simulink model "controller_for_bicycle"  (R2021a)
settings: Solver=VariableStepAuto  StartTime=0.0  StopTime=10.0  RelTol=1e-3
values from neighbouring files (symbols this model uses):
  Fyf = zeros(1,57)    [FyfLookUpNewCar.m]    (also in Fyf_loopup_table.mat = [-9372.31873381 -9371.87234491 -9368.75632133 -9360.32413915)
  SlipAngle = -SlipAngle    [FyfLookUpNewCar.m]    (also in Fyf_loopup_table.mat = [0.153111393254 0.147643129209 0.142174865164 0.13670660112 )
libraries: simulink_extras x1, autolibshared x1, simulink x1
settings Model: Creator=chnwa  LastModifiedBy=chnwa

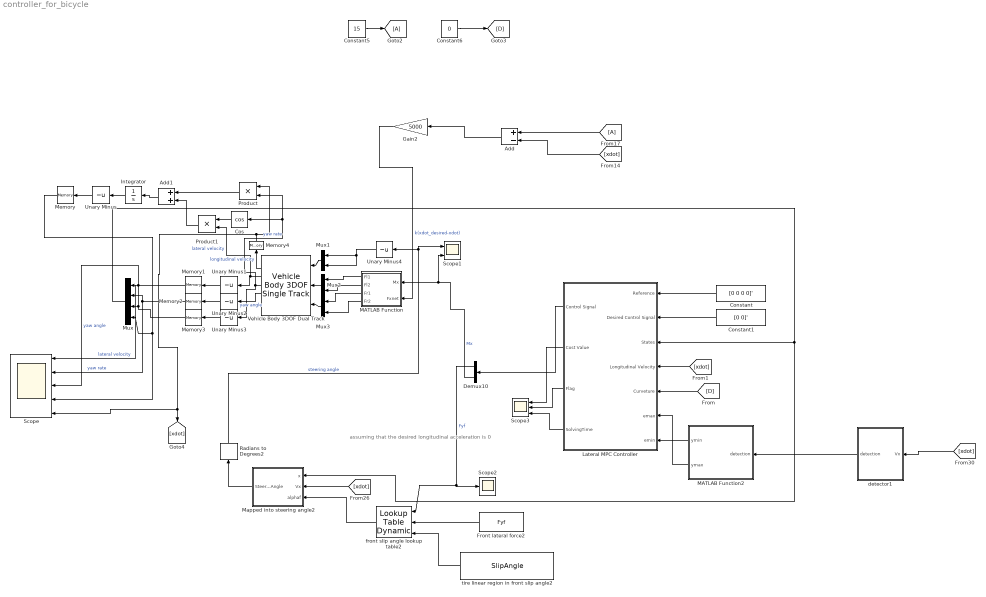
== system controller_for_bicycle ==
  note: assuming that the desired longitudinal acceleration is 0
  Add : Sum  Inputs=+-
  Add1 : Sum
  Constant : Constant  Value=[0 0 0 0]'
  Constant1 : Constant  Value=[0 0]'
  Constant5 : Constant  Value=15
  Constant6 : Constant  Value=0
  Cos : Trigonometry  Operator=cos
  Demux10 : Demux  Outputs=2
  Front lateral force2 : Constant  Value=Fyf
  Gain2 : Gain  Gain=5000
  Integrator : Integrator
  Lateral MPC Controller : Subsystem
  MATLAB Function : MATLAB Function  TreatAsAtomicUnit=on
  MATLAB Function2 : MATLAB Function  TreatAsAtomicUnit=on
  Mapped into steering angle2 : MATLAB Function  TreatAsAtomicUnit=on
  Memory{,1..3} (4 alike) : Memory
  Memory4 : Memory  InitialCondition=15
  Mux : Mux
  Mux1 : Mux  Inputs=2
  Mux2 : Mux  Inputs=2
  Mux3 : Mux  Inputs=2
  Product : Product
  Product1 : Product
  Radians to Degrees2 : simulink_extras/Transformations/Radians to Degrees
  Scope : Scope  NumInputPorts=5
  Scope1 : Scope  NumInputPorts=2
  Scope2 : Scope
  Scope3 : Scope  NumInputPorts=3
  Unary Minus{,1..4} (5 alike) : UnaryMinus
  Vehicle Body 3DOF Dual Track : autolibshared/Vehicle Body 3DOF Single Track  trackMode=Dual  inputMode=External longitudinal forces  frontSteerMode=on  rearSteerMode=off  windMode=off  muMode=off  extFMode=off  extMMode=off  htchFMode=off  htchMMode=off  extXo=off  extpsio=off  extxdoto=off  extro=off  extYo=off  extTamb=off  extydoto=off  aMode=2  NF=2  NR=2  m=2272  a=1.11  b=1.67  h=0.35  dh=1  hh=0.2  X_o=0  xdot_o=15  CalphaMode=off  sigmaMode=on  d=0  hl=0  w=[1.4,1.4]  Cy_f=1.822e5  Cy_r=1.822e5  sigma_f=.1  sigma_r=.1  alpha_f_brk=[-.1 .1]  Cy_f_data=[-9e3 9e3]  alpha_r_brk=[-.1 .1]  Cy_r_data=[-9e3 9e3]  Y_o=0  ydot_o=0  Izz=4600  psi_o=0  r_o=0  Af=2  Cd=.3  Cl=.1  Cpm=.1  beta_w=[0:0.01:0.3]  Cs=[0:0.03:0.9]  Cym=[0:0.01:0.3]  Pabs=101325  Tair=273  g=9.81  mu=0.7  xdot_tol=.01  Fznom=5000  Fxtire_sat=7e4  Fytire_sat=7e4  longOff=0  latOff=0  vertOff=0  wrapAng=off
      settings: SourceProductBaseCode=PW,DR,MT,UV,VE
  detector1 : Subsystem
  front slip angle lookup table2 : simulink/Lookup Tables/Lookup Table Dynamic  LookUpMeth=Interpolation-Use End Values  OutDataType=fixdt('double')  OutScaling=[]  OutputDataTypeScalingMode=Specify via dialog  OutDataTypeStr=double  DoSatur=off
  tire linear region in front slip angle2 : Constant  Value=SlipAngle
  wires:
  [xdot] -> Lateral MPC Controller/4(Longitudinal Velocity)
  tire linear region in front slip angle2/1 -> front slip angle lookup table2/3
  Memory3/1 -> Scope/3, Mux/3  "yaw angle"
  Constant/1 -> Lateral MPC Controller/1(Reference)
  Lateral MPC Controller/2(Cost Value) -> Scope3/1
  MATLAB Function/3(Fr1) -> Mux3/1
  [xdot] -> detector1/1(Vx)
  MATLAB Function2/2(ymax) -> Lateral MPC Controller/6(emax)
  Lateral MPC Controller/4(SolvingTime) -> Scope3/3
  front slip angle lookup table2/1 -> Mapped into steering angle2/3(alphaf)
  Lateral MPC Controller/3(Flag) -> Scope3/2
  Demux10/2 -> Scope1/2, MATLAB Function/1(Mx)  "Mx"
  Lateral MPC Controller/1(Control Signal) -> Demux10/1
  MATLAB Function/1(Fl1) -> Mux2/1
  MATLAB Function/2(Fl2) -> Mux2/2
  MATLAB Function/4(Fr2) -> Mux3/2
  Demux10/1 -> Scope2/1, front slip angle lookup table2/1  "Fyf"
  Gain2/1 -> MATLAB Function/2(Fxnet)  "k(xdot_desired-xdot)"
  Mux/1 -> Mapped into steering angle2/1(x), Lateral MPC Controller/3(States)
  [A] -> Add/1
  Radians to Degrees2/1 -> Unary Minus4/1, Scope1/1  "steering angle"
  [D] -> Lateral MPC Controller/5(Curveture)
  Memory2/1 -> Scope/2, Mux/2  "yaw rate"
  Mapped into steering angle2/1(SteeringAngle) -> Radians to Degrees2/1
  MATLAB Function2/1(ymin) -> Lateral MPC Controller/7(emin)
  [xdot] -> Mapped into steering angle2/2(Vx)
  [xdot] -> Add/2
  Front lateral force2/1 -> front slip angle lookup table2/2
  detector1/1(detection) -> MATLAB Function2/1(detection)
  Vehicle Body 3DOF Dual Track/2 -> Memory4/1  "longitudinal velocity"
  Add/1 -> Gain2/1
  Memory1/1 -> Scope/1, Mux/1  "lateral velocity"
  Constant1/1 -> Lateral MPC Controller/2(Desired Control Signal)
  Mux1/1 -> Vehicle Body 3DOF Dual Track/1
  Mux2/1 -> Vehicle Body 3DOF Dual Track/2
  Mux3/1 -> Vehicle Body 3DOF Dual Track/3
  Unary Minus/1 -> Memory/1
  Memory/1 -> Scope/4, Mux/4
  Unary Minus1/1 -> Memory1/1
  Vehicle Body 3DOF Dual Track/3 -> Product1/2, Unary Minus1/1  "lateral velocity"
  Unary Minus2/1 -> Memory2/1
  Vehicle Body 3DOF Dual Track/5 -> Unary Minus2/1  "yaw angle"
  Unary Minus3/1 -> Memory3/1
  Vehicle Body 3DOF Dual Track/4 -> Product/2, Cos/1, Unary Minus3/1  "yaw rate"
  Unary Minus4/1 -> Mux1/2, Mux1/1
  Constant5/1 -> [A]
  Constant6/1 -> [D]
  Cos/1 -> Product1/1
  Product/1 -> Add1/1
  Product1/1 -> Add1/2
  Add1/1 -> Integrator/1
  Integrator/1 -> Unary Minus/1
  Memory4/1 -> Product/1, [xdot], Scope/5

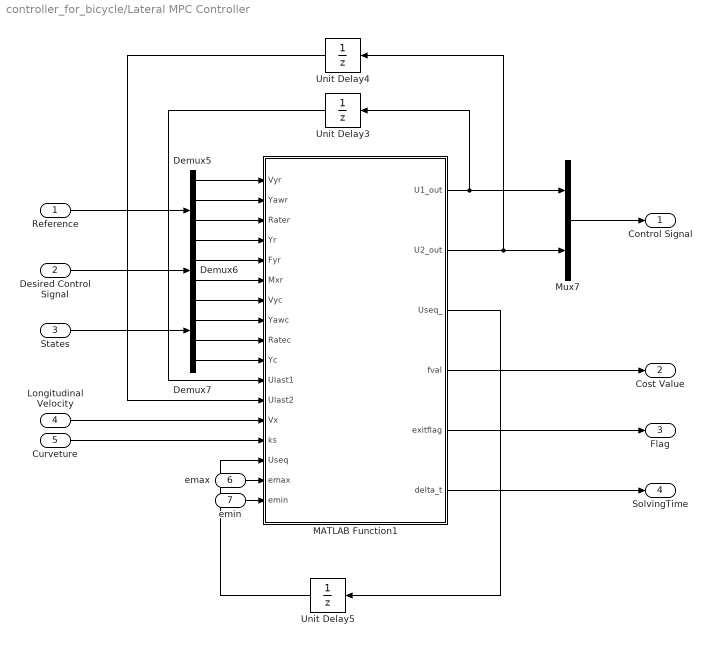
== system controller_for_bicycle/Lateral MPC Controller ==
  Reference : Inport
  Desired Control Signal : Inport  Port=2
  States : Inport  Port=3
  Longitudinal Velocity : Inport  Port=4
  Curveture : Inport  Port=5
  emax : Inport  Port=6
  emin : Inport  Port=7
  Demux5 : Demux
  Demux6 : Demux  Outputs=2
  Demux7 : Demux
  MATLAB Function1 : MATLAB Function  TreatAsAtomicUnit=on
  Mux7 : Mux  Inputs=2
  Unit Delay3 : UnitDelay  SampleTime=-1  HasFrameUpgradeWarning=on
  Unit Delay4 : UnitDelay  SampleTime=-1  HasFrameUpgradeWarning=on
  Unit Delay5 : UnitDelay  InitialCondition=zeros(31,2)  SampleTime=-1  HasFrameUpgradeWarning=on
  Control Signal : Outport
  Cost Value : Outport  Port=2
  Flag : Outport  Port=3
  SolvingTime : Outport  Port=4
  wires:
  Demux5/3 -> MATLAB Function1/3(Rater)
  Desired Control Signal/1 -> Demux6/1
  MATLAB Function1/5(exitflag) -> Flag/1
  MATLAB Function1/2(U2_out) -> Mux7/2, Unit Delay4/1
  Demux5/1 -> MATLAB Function1/1(Vyr)
  Unit Delay4/1 -> MATLAB Function1/12(Ulast2)
  Longitudinal Velocity/1 -> MATLAB Function1/13(Vx)
  Demux7/3 -> MATLAB Function1/9(Ratec)
  MATLAB Function1/3(Useq_) -> Unit Delay5/1
  Demux7/1 -> MATLAB Function1/7(Vyc)
  Demux5/4 -> MATLAB Function1/4(Yr)
  MATLAB Function1/4(fval) -> Cost Value/1
  Curveture/1 -> MATLAB Function1/14(ks)
  emax/1 -> MATLAB Function1/16(emax)
  MATLAB Function1/1(U1_out) -> Mux7/1, Unit Delay3/1
  Demux7/2 -> MATLAB Function1/8(Yawc)
  Demux7/4 -> MATLAB Function1/10(Yc)
  Reference/1 -> Demux5/1
  Mux7/1 -> Control Signal/1
  Unit Delay5/1 -> MATLAB Function1/15(Useq)
  Unit Delay3/1 -> MATLAB Function1/11(Ulast1)
  States/1 -> Demux7/1
  MATLAB Function1/6(delta_t) -> SolvingTime/1
  Demux6/2 -> MATLAB Function1/6(Mxr)
  Demux6/1 -> MATLAB Function1/5(Fyr)
  Demux5/2 -> MATLAB Function1/2(Yawr)
  emin/1 -> MATLAB Function1/17(emin)

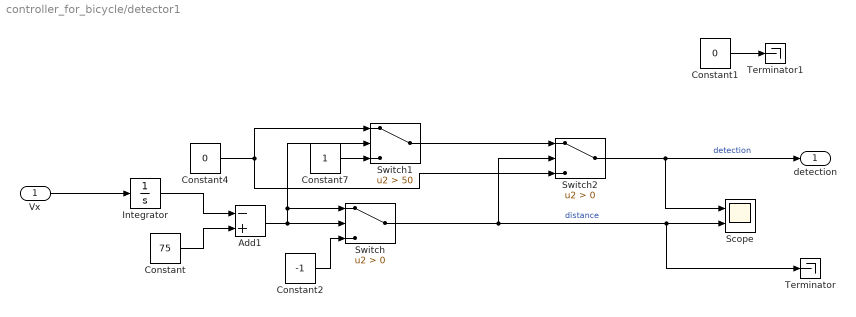
== system controller_for_bicycle/detector1 ==
  Vx : Inport
  Add1 : Sum  Inputs=-+
  Constant : Constant  Value=75
  Constant1 : Constant  Value=0
  Constant2 : Constant  Value=-1
  Constant4 : Constant  Value=0
  Constant7 : Constant
  Integrator : Integrator
  Scope : Scope  NumInputPorts=2
  Switch : Switch  Criteria=u2 > Threshold
  Switch1 : Switch  Criteria=u2 > Threshold  Threshold=50
  Switch2 : Switch  Criteria=u2 > Threshold
  Terminator : Terminator
  Terminator1 : Terminator
  detection : Outport
  wires:
  Constant2/1 -> Switch/3
  Constant4/1 -> Switch2/3, Switch1/1
  Vx/1 -> Integrator/1
  Integrator/1 -> Add1/1
  Switch/1 -> Switch2/2, Terminator/1, Scope/2  "distance"
  Constant7/1 -> Switch1/3
  Add1/1 -> Switch1/2, Switch/1, Switch/2
  Switch1/1 -> Switch2/1
  Constant/1 -> Add1/2
  Switch2/1 -> detection/1, Scope/1  "detection"
  Constant1/1 -> Terminator1/1

== matlab function controller_for_bicycle/MATLAB Function2 ==
  data: detection input; ymin output; ymax output
function [ymin,ymax] = fcn(detection)

% miu = 0.7; %frction cooeficient 0.7 for dry road and 0.4 for wet
% g = 9.81; % gravity
% m = 2272;   %mass
% lf = 1.11;  % distance from front axle to the mass center
% lr = 1.67;  % distance from rear axle to the mass center
% C_a = 1.822e5; % rear cornering stifness
% 
% Fz = m*g*lf/(lf+lr)/2; % the load that beared by the rear tire
% 
% rmax = g*miu/Vx; %max yaw rate
% threshold = atan(3*miu*Fz/C_a);
% 
% r = x(2);
% vmax = lr*r+Vx*threshold;   %max lateral velocity
% vmin = lr*r-Vx*threshold;   %min lateral velocity

if detection == 1
    ymin = 5;%50m is the distance from which obstacle is detected
    ymax = 10;
else
    ymin = -10;
    ymax = 10;
end

== matlab function controller_for_bicycle/Lateral MPC Controller/MATLAB Function1 ==
  data: Vyr input; U1_out output; Yawr input; Rater input; Yr input; Fyr input; Mxr input; Vyc input; Yawc input; Ratec input; Yc input; Ulast1 input; Ulast2 input; Vx input; ks input; Useq input; U2_out output; Useq_ output; fval output; exitflag output; delta_t output; emax input; emin input
function [U1_out,U2_out,Useq_,fval,exitflag,delta_t] = fcn(Vyr,Yawr,Rater,Yr, Fyr,Mxr,Vyc,Yawc,Ratec,Yc,Ulast1,Ulast2,Vx,ks,Useq,emax,emin)
%Vyr lateral velocity, Yawr yaw angle, Rater yaw rate, Yr lateral position
%Fyr lateral force in front tyre,Mxr moment generated by longitudinal force
%'r'means reference ||  'c'means current
    lr=1.67;
    threshold=0.213;
    miu=0.7;
    rmax=9.81*miu/Vx;
%% Initilization    
    tstart=tic;%timing on
    
    Nx=4;%number of state
    Nu=2;%number of control
    Np=30;%prediction horizon
    Nc=1;%control horizon

    %reference
    r=zeros(Nx,1);%state reference
    r(1)=Vyr;
    r(2)=Yawr;
    r(3)=Rater;
    r(4)=Yr;    
    ur1=Fyr;
    ur2=Mxr;%control reference
    
    %states
    x=zeros(Nx,1);%state reference
    x(1)=Vyc;
    x(2)=Yawc;
    x(3)=Ratec;
    x(4)=Yc;   
    
    %control
    u=zeros(Nu,1);%state reference
    u(1)=Ulast1;
    u(2)=Ulast2;
    
    %get augmented states
    kesi=zeros(Nx+Nu,1);%[X;U]
    kesi(1)=x(1)-r(1);
    kesi(2)=x(2)-r(2);
    kesi(3)=x(3)-r(3);
    kesi(4)=x(4)-r(4);
    kesi(5)=u(1);
    kesi(6)=u(2);
    
    Ts=0.1;%sample time
    
%% Modellng->Discretization->prediction->quadratic programming
    %Modelling&Linearization&Discretization
    steps=Np+1;
    A = zeros(Nx+Nu,Nx+Nu,steps);
    B = zeros(Nx+Nu,Nu,steps);
    Dc = zeros(Nx,1,steps);
    C=[1 0 0 0 0 0;0 1 0 0 0 0;0 0 1 0 0 0;0 0 0 1 0 0];
    
    for ct = 1:steps
        if ct>length(Useq)
            uk = Useq(Np,:);
        else
            uk = Useq(ct,:);
        end
        uk=uk';
        [Ad, Bd, DK, delta_x] = GetDynamics(Vx,ks,x,uk,Ts);
        A(:,:,ct)=[Ad,Bd;zeros(Nu,Nx),eye(Nu)];        
        B(:,:,ct)=[Bd;ones(Nu,Nu)];
        Dc(:,:,ct)=DK;
        x=x+delta_x;    
    end
    %construct important matrix
    coder.varsize('PHI',[Np*Nx,Nx+Nu]);
    coder.varsize('THETA',[Np*Nx,Nc*Nu]);
    coder.varsize('D',[Np*Nx,1]);
    PHI=[];
    THETA=[];
    D=[];
    product=eye(6);
    for j=1:Np
        product=A(:,:,j)*product;
        PHI=[PHI;C*product];
        D=[D;Dc(:,:,j)];
    end
    for k=1:Nc
        product1=eye(6);
        for j=1:Np
            THETA=[THETA;C*product1*B(:,:,k)];
            product1=A(:,:,j+1)*product1;
        end
    end
    Sigma=zeros(Np,Nc);
    for p=1:Np%define a lower triangular matrix
        for q=1:1:Nc
            if q<=p 
                Sigma(p,q)=1;
            else 
                Sigma(p,q)=0;
            end
        end 
    end 
    UT=kron(ones(Np,1),[u(1);u(2)]);
    Sigma=kron(Sigma,ones(Nu,Nu));
    error=PHI*kesi;
    Q=kron(eye(Np,Np),diag([0 0 100 4]));    
    R=kron(eye(Np,Np),diag([0 4e-5]));    
    P=diag([3e-5 8e-5]);
    rou1=3e3;    
    rou2=5e4;
    H=2*[THETA'*Q*THETA+Sigma'*R*Sigma+P zeros(2,2);0 0 rou1 0;0 0 0 rou2];%是否要乘2？要
    f=[2*(error'*Q*THETA+D'*Q*THETA+UT'*R*Sigma),0,0];%是否要转置？好像无所谓
   %% constraints
    %inequation
    A_t=zeros(Nc,Nc);
    for p=1:1:Nc%define a lower triangular matrix
        for q=1:1:Nc
            if q<=p 
                A_t(p,q)=1;
            else 
                A_t(p,q)=0;
            end
        end 
    end 
    A_I=kron(A_t,eye(Nu)); 
    Ut=kron(ones(Nc,1),[Ulast1;Ulast2]);%control in last control step
    umin=[-1e4; -1e3];
    umax=[1e4; 1e3];
    Umin=kron(ones(Nc,1),umin);
    Umax=kron(ones(Nc,1),umax);
    coder.varsize('A_cons',[Np*6+4,4]);
    coder.varsize('b_cons',[Np*6+4,1]);
    A_cons=[A_I zeros(Nu*Nc,2);-A_I zeros(Nu*Nc,2)];
    b_cons=[Umax-Ut;-Umin+Ut];
    %add handling envelop constriants & environment envolop
    gamas=[1 -lr 0 0;-1 lr 0 0;0 1 0 0;0 -1 0 0];
    gamae=[0 0 0 1;0 0 0 -1];
    for i=1:4:Np
        Gs=[Vx*threshold;Vx*threshold;rmax;rmax];
        A_cons=[A_cons;[gamas*THETA(i:i+3,:) -ones(4,1) zeros(4,1)];[gamae*THETA(i:i+3,:) zeros(2,1) -ones(2,1)]];
        b_cons=[b_cons;[Gs-gamas*PHI(i:i+3,:)*kesi];[emax;-emin]-gamae*PHI(i:i+3,:)*kesi];
    end
    
    %upper and lower boundary
    delta_umin=[-1e4;-1e3];
    delta_umax=[1e4;1e3];
    M1=10; %related to slack variable
    M2=10; %related to slack variable
    delta_Umin=kron(ones(Nc,1),delta_umin);
    delta_Umax=kron(ones(Nc,1),delta_umax);
    lb=[delta_Umin;0;0];
    ub=[delta_Umax;M1;M2];  
   %% solve quadratic programming
    opts = optimoptions('quadprog','Algorithm','active-set');
    x_start=zeros(Nu*Nc+2,1);%+2 corresponds to slack variables
    [X,fval,exitflag]=quadprog(H,f',A_cons,b_cons,[],[],lb,ub,x_start,opts);
    
   %% calculate control signal
    U1=kesi(5)+X(1);%The output error at the previous time plus the optimization result to get the error at this time
    U2=kesi(6)+X(2);%The output error at the previous time plus the optimization result to get the error at this time
    U1_out=U1+ur1;%Error plus reference value to get final output value    
    U2_out=U2+ur2;
    delta_t=toc(tstart);%timing off
    Useq_=repmat([U1,U2],Np+1,1);
end

function [A, B, DK, delta_x] = GetDynamics(Vx,ks,x,u,Ts)

%Plant Model parameters
m = 2272;   %mass
Iz = 4600;  %rotational inertia
lf = 1.11;  % distance from front axle to the mass center
lr = 1.67;  % distance from rear axle to the mass center
C_a = 1.822e5; % rear cornering stiffness 

%Enviroment parameters
miu = 0.7; %frction cooeficient 0.7 for dry road and 0.4 for wet
g = 9.81; % gravity

Fz = m*g*lf/(lf+lr)/2; % the load that beared by the rear tire

%calculate alpha
Vy = x(1); %lateral velocity
r = x(2);  %yaw rate
alphar_ = Vy/Vx-lr*r/Vx;   %calculate linearzing point

%tire model
threshold = atan(3*miu*Fz/C_a);     % threshold for the tire linear region
if abs(alphar_)<threshold
    %the rear lateral force value (f(x0)) at the linearzing point
    Fyr_ = -C_a*tan(alphar_)+C_a^2/(3*miu*Fz)*abs(tan(alphar_))*tan(alphar_)-C_a^3/(27*miu^2*Fz^2)*tan(alphar_)^3;
    
    %the slope of linearized model (f‘(x0))
    if alphar_>= 0
        Cr_ = -C_a*sec(alphar_)^2+C_a^2/(3*miu*Fz)*(2*sec(alphar_)^2*tan(alphar_))-C_a^3/(27*miu^2*Fz^2)*(3*tan(alphar_)^2*sec(alphar_)^2);
    else
        Cr_ = -C_a*sec(alphar_)^2-C_a^2/(3*miu*Fz)*(2*sec(alphar_)^2*tan(alphar_))-C_a^3/(27*miu^2*Fz^2)*(3*tan(alphar_)^2*sec(alphar_)^2);
    end
else
    
    %the saturation region of tire model
    Fyr_ = -miu*Fz*sign(alphar_);
    Cr_ = 0;
end

%Continuous-time model
Ac = [Cr_/(m*Vx) -lr*Cr_/(m*Vx)-Vx 0 0;
    -lr*Cr_/(Iz*Vx) lr^2*Cr_/(Iz*Vx) 0 0;
    0 1 0 0;
    1 0 Vx 0];
Bc = [1/m 0;
    lf/Iz 1/Iz;
    0 0;
    0 0];
dcc = [(Fyr_-Cr_*alphar_)/m;
    -lr*(Fyr_-Cr_*alphar_)/Iz;
    -Vx*ks;
    0];

G=[Ac Bc dcc;zeros(3,7)];
M=expm(G*Ts);
A=M(1:4,1:4);
B=M(1:4,5:6);
DK=M(1:4,7);
delta_x=A*x+B*u+DK-x;
end

== matlab function controller_for_bicycle/Mapped into steering angle2 ==
  data: x input; Vx input; alphaf input; SteeringAngle output
function SteeringAngle = fcn(x,Vx, alphaf)

lf = 1.11;  % distance from front axle to the mass center

Vy = x(1); %lateral velocity
r = x(2);  %yaw rate
SteeringAngle = Vy/Vx+lf*r/Vx-alphaf;

== matlab function controller_for_bicycle/MATLAB Function ==
  data: Fl1 output; Mx input; Fl2 output; Fxnet input; Fr1 output; Fr2 output
function [Fl1,Fl2,Fr1,Fr2] = fcn(Mx,Fxnet)

w = 1.875; % the width of the car

Fwf = zeros(2,1);
Fwr = zeros(2,1);

if Mx > 0
    Fwf(1) = Fxnet/2-Mx/w;
    Fwf(2) = Fxnet/2;
    Fwr(1) = -Mx/w;
    Fwr(2) = 0;
elseif Mx < 0
    Fwf(1) = Fxnet/2;
    Fwf(2) = Fxnet/2+Mx/w;
    Fwr(1) = 0;
    Fwr(2) = Mx/w;
else
    Fwf(1) = Fxnet/2+0;
    Fwf(2) = Fxnet/2+0;
    Fwr(1) = 0;
    Fwr(2) = 0;
end
Fl1 = Fwf(1);
Fl2 = Fwr(1);
Fr1 = Fwf(2);
Fr2 = Fwr(2);
